simulink model "DSSDK_TrackerMultipleObject"  (Simulink 8.4)
settings: Solver=FixedStepDiscrete  StartTime=0.0  StopTime=inf  RelTol=1e-3
settings Model: Creator=Ssubrama  LastModifiedBy=kpetersen
settings OptimizationCC: InitFltsAndDblsToZero=on
settings GRTTargetCC: TargetFcnLib=ansi_tfl_tmw_new.mat

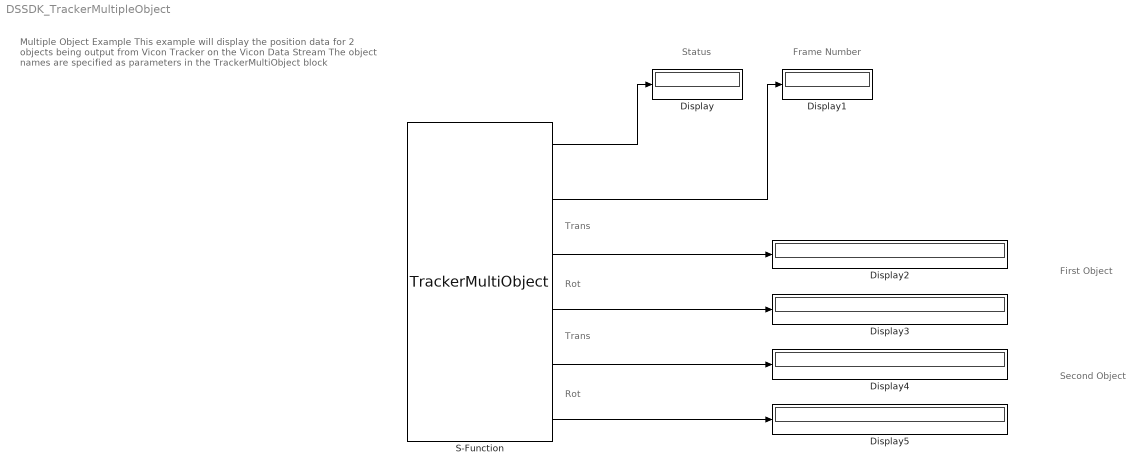
== system DSSDK_TrackerMultipleObject ==
  note: Multiple Object Example
      |
      | This example will display the position data
      | for 2 objects being output from
      | Vicon Tracker on the Vicon Data Stream
      |
      | The object names are specified as parameters
      | in the TrackerMultiObject block
  note: Frame Number
  note: Status
  note: First Object
  note: Second Object
  note: Trans
  note: Trans
  note: Rot
  note: Rot
  Display{,1..5} (6 alike) : Display
      Display settings: Format=hex (Stored Integer)
  S-Function : S-Function  FunctionName=TrackerMultiObject  Parameters='Object1','Object2'  SFunctionModules=TrackerMultiObject  EnableBusSupport=off
      settings: AttributesFormatString=Data Parser
  wires:
  S-Function/1 -> Display/1
  S-Function/2 -> Display1/1
  S-Function/3 -> Display2/1
  S-Function/4 -> Display3/1
  S-Function/5 -> Display4/1
  S-Function/6 -> Display5/1
